simulink model "ARAI_Academy"  (R2020a)
settings: Solver=FixedStepDiscrete  StartTime=0.0  StopTime=10.0  FixedStep=0.02  RelTol=1e-3
InitFcn:
  | mbd_s32k_consistency_checks(bdroot(gcs));
undefined symbols (not defined in the file): Cells_in_Series, LQFP, Temp_in_Series, ts
libraries: hdlsllib x280, mbd_s32k1xx_ec_toolbox x39, simulink x3
(part 3 of 3)

== system ARAI_Academy/Subsystem15/Subsystem12/Subsystem8 ==
  u : Inport
  Bit Slice : hdlsllib/Logic and Bit Operations/Bit Slice  lidx=15  ridx=8
      settings: SourceProductBaseCode=SL
  Bit Slice1 : hdlsllib/Logic and Bit Operations/Bit Slice  lidx=7  ridx=0
      settings: SourceProductBaseCode=SL
  Mux : Mux  Inputs=2
  Out1 : Outport
  wires:
  Bit Slice/1 -> Mux/1
  u/1 -> Bit Slice/1, Bit Slice1/1
  Bit Slice1/1 -> Mux/2
  Mux/1 -> Out1/1

== system ARAI_Academy/Subsystem16/Subsystem12/Subsystem ==
  u : Inport
  Bit Slice : hdlsllib/Logic and Bit Operations/Bit Slice  lidx=15  ridx=8
      settings: SourceProductBaseCode=SL
  Bit Slice1 : hdlsllib/Logic and Bit Operations/Bit Slice  lidx=7  ridx=0
      settings: SourceProductBaseCode=SL
  Mux : Mux  Inputs=2
  Out1 : Outport
  wires:
  Bit Slice/1 -> Mux/1
  u/1 -> Bit Slice/1, Bit Slice1/1
  Bit Slice1/1 -> Mux/2
  Mux/1 -> Out1/1

== system ARAI_Academy/Subsystem16/Subsystem12/Subsystem1 ==
  u : Inport
  Bit Slice : hdlsllib/Logic and Bit Operations/Bit Slice  lidx=15  ridx=8
      settings: SourceProductBaseCode=SL
  Bit Slice1 : hdlsllib/Logic and Bit Operations/Bit Slice  lidx=7  ridx=0
      settings: SourceProductBaseCode=SL
  Mux : Mux  Inputs=2
  Out1 : Outport
  wires:
  Bit Slice/1 -> Mux/1
  u/1 -> Bit Slice/1, Bit Slice1/1
  Bit Slice1/1 -> Mux/2
  Mux/1 -> Out1/1

== system ARAI_Academy/Subsystem16/Subsystem12/Subsystem2 ==
  u : Inport
  Bit Slice : hdlsllib/Logic and Bit Operations/Bit Slice  lidx=15  ridx=8
      settings: SourceProductBaseCode=SL
  Bit Slice1 : hdlsllib/Logic and Bit Operations/Bit Slice  lidx=7  ridx=0
      settings: SourceProductBaseCode=SL
  Mux : Mux  Inputs=2
  Out1 : Outport
  wires:
  Bit Slice/1 -> Mux/1
  u/1 -> Bit Slice/1, Bit Slice1/1
  Bit Slice1/1 -> Mux/2
  Mux/1 -> Out1/1

== system ARAI_Academy/Subsystem16/Subsystem12/Subsystem3 ==
  u : Inport
  Bit Slice : hdlsllib/Logic and Bit Operations/Bit Slice  lidx=15  ridx=8
      settings: SourceProductBaseCode=SL
  Bit Slice1 : hdlsllib/Logic and Bit Operations/Bit Slice  lidx=7  ridx=0
      settings: SourceProductBaseCode=SL
  Mux : Mux  Inputs=2
  Out1 : Outport
  wires:
  Bit Slice/1 -> Mux/1
  u/1 -> Bit Slice/1, Bit Slice1/1
  Bit Slice1/1 -> Mux/2
  Mux/1 -> Out1/1

== system ARAI_Academy/Subsystem16/Subsystem12/Subsystem4 ==
  u : Inport
  Bit Slice : hdlsllib/Logic and Bit Operations/Bit Slice  lidx=15  ridx=8
      settings: SourceProductBaseCode=SL
  Bit Slice1 : hdlsllib/Logic and Bit Operations/Bit Slice  lidx=7  ridx=0
      settings: SourceProductBaseCode=SL
  Mux : Mux  Inputs=2
  Out1 : Outport
  wires:
  Bit Slice/1 -> Mux/1
  u/1 -> Bit Slice/1, Bit Slice1/1
  Bit Slice1/1 -> Mux/2
  Mux/1 -> Out1/1

== system ARAI_Academy/Subsystem16/Subsystem12/Subsystem5 ==
  u : Inport
  Bit Slice : hdlsllib/Logic and Bit Operations/Bit Slice  lidx=15  ridx=8
      settings: SourceProductBaseCode=SL
  Bit Slice1 : hdlsllib/Logic and Bit Operations/Bit Slice  lidx=7  ridx=0
      settings: SourceProductBaseCode=SL
  Mux : Mux  Inputs=2
  Out1 : Outport
  wires:
  Bit Slice/1 -> Mux/1
  u/1 -> Bit Slice/1, Bit Slice1/1
  Bit Slice1/1 -> Mux/2
  Mux/1 -> Out1/1

== system ARAI_Academy/Subsystem16/Subsystem12/Subsystem7 ==
  u : Inport
  Bit Slice : hdlsllib/Logic and Bit Operations/Bit Slice  lidx=15  ridx=8
      settings: SourceProductBaseCode=SL
  Bit Slice1 : hdlsllib/Logic and Bit Operations/Bit Slice  lidx=7  ridx=0
      settings: SourceProductBaseCode=SL
  Mux : Mux  Inputs=2
  Out1 : Outport
  wires:
  Mux/1 -> Out1/1
  Bit Slice1/1 -> Mux/2
  u/1 -> Bit Slice1/1, Bit Slice/1
  Bit Slice/1 -> Mux/1

== system ARAI_Academy/Subsystem16/Subsystem12/Subsystem8 ==
  u : Inport
  Bit Slice : hdlsllib/Logic and Bit Operations/Bit Slice  lidx=15  ridx=8
      settings: SourceProductBaseCode=SL
  Bit Slice1 : hdlsllib/Logic and Bit Operations/Bit Slice  lidx=7  ridx=0
      settings: SourceProductBaseCode=SL
  Mux : Mux  Inputs=2
  Out1 : Outport
  wires:
  Bit Slice/1 -> Mux/1
  u/1 -> Bit Slice/1, Bit Slice1/1
  Bit Slice1/1 -> Mux/2
  Mux/1 -> Out1/1

== system ARAI_Academy/Subsystem9/Subsystem/Subsystem ==
  u : Inport
  Bit Slice : hdlsllib/Logic and Bit Operations/Bit Slice  lidx=15  ridx=8
      settings: SourceProductBaseCode=SL
  Bit Slice1 : hdlsllib/Logic and Bit Operations/Bit Slice  lidx=7  ridx=0
      settings: SourceProductBaseCode=SL
  Mux : Mux  Inputs=2
  Out1 : Outport
  wires:
  Bit Slice/1 -> Mux/1
  u/1 -> Bit Slice/1, Bit Slice1/1
  Bit Slice1/1 -> Mux/2
  Mux/1 -> Out1/1

== system ARAI_Academy/Subsystem9/Subsystem/Subsystem1 ==
  u : Inport
  Bit Slice : hdlsllib/Logic and Bit Operations/Bit Slice  lidx=15  ridx=8
      settings: SourceProductBaseCode=SL
  Bit Slice1 : hdlsllib/Logic and Bit Operations/Bit Slice  lidx=7  ridx=0
      settings: SourceProductBaseCode=SL
  Mux : Mux  Inputs=2
  Out1 : Outport
  wires:
  Bit Slice/1 -> Mux/1
  u/1 -> Bit Slice/1, Bit Slice1/1
  Bit Slice1/1 -> Mux/2
  Mux/1 -> Out1/1

== system ARAI_Academy/Subsystem9/Subsystem/Subsystem10 ==
  u : Inport
  Bit Slice : hdlsllib/Logic and Bit Operations/Bit Slice  lidx=15  ridx=8
      settings: SourceProductBaseCode=SL
  Bit Slice1 : hdlsllib/Logic and Bit Operations/Bit Slice  lidx=7  ridx=0
      settings: SourceProductBaseCode=SL
  Mux : Mux  Inputs=2
  Out1 : Outport
  wires:
  Bit Slice/1 -> Mux/1
  u/1 -> Bit Slice/1, Bit Slice1/1
  Bit Slice1/1 -> Mux/2
  Mux/1 -> Out1/1

== system ARAI_Academy/Subsystem9/Subsystem/Subsystem11 ==
  u : Inport
  Bit Slice : hdlsllib/Logic and Bit Operations/Bit Slice  lidx=15  ridx=8
      settings: SourceProductBaseCode=SL
  Bit Slice1 : hdlsllib/Logic and Bit Operations/Bit Slice  lidx=7  ridx=0
      settings: SourceProductBaseCode=SL
  Mux : Mux  Inputs=2
  Out1 : Outport
  wires:
  Mux/1 -> Out1/1
  Bit Slice1/1 -> Mux/2
  u/1 -> Bit Slice1/1, Bit Slice/1
  Bit Slice/1 -> Mux/1

== system ARAI_Academy/Subsystem9/Subsystem/Subsystem12 ==
  u : Inport
  Bit Slice : hdlsllib/Logic and Bit Operations/Bit Slice  lidx=15  ridx=8
      settings: SourceProductBaseCode=SL
  Bit Slice1 : hdlsllib/Logic and Bit Operations/Bit Slice  lidx=7  ridx=0
      settings: SourceProductBaseCode=SL
  Mux : Mux  Inputs=2
  Out1 : Outport
  wires:
  Bit Slice/1 -> Mux/1
  u/1 -> Bit Slice/1, Bit Slice1/1
  Bit Slice1/1 -> Mux/2
  Mux/1 -> Out1/1

== system ARAI_Academy/Subsystem9/Subsystem/Subsystem13 ==
  u : Inport
  Bit Slice : hdlsllib/Logic and Bit Operations/Bit Slice  lidx=15  ridx=8
      settings: SourceProductBaseCode=SL
  Bit Slice1 : hdlsllib/Logic and Bit Operations/Bit Slice  lidx=7  ridx=0
      settings: SourceProductBaseCode=SL
  Mux : Mux  Inputs=2
  Out1 : Outport
  wires:
  Mux/1 -> Out1/1
  Bit Slice1/1 -> Mux/2
  u/1 -> Bit Slice1/1, Bit Slice/1
  Bit Slice/1 -> Mux/1

== system ARAI_Academy/Subsystem9/Subsystem/Subsystem14 ==
  u : Inport
  Bit Slice : hdlsllib/Logic and Bit Operations/Bit Slice  lidx=15  ridx=8
      settings: SourceProductBaseCode=SL
  Bit Slice1 : hdlsllib/Logic and Bit Operations/Bit Slice  lidx=7  ridx=0
      settings: SourceProductBaseCode=SL
  Mux : Mux  Inputs=2
  Out1 : Outport
  wires:
  Bit Slice/1 -> Mux/1
  u/1 -> Bit Slice/1, Bit Slice1/1
  Bit Slice1/1 -> Mux/2
  Mux/1 -> Out1/1

== system ARAI_Academy/Subsystem9/Subsystem/Subsystem15 ==
  u : Inport
  Bit Slice : hdlsllib/Logic and Bit Operations/Bit Slice  lidx=15  ridx=8
      settings: SourceProductBaseCode=SL
  Bit Slice1 : hdlsllib/Logic and Bit Operations/Bit Slice  lidx=7  ridx=0
      settings: SourceProductBaseCode=SL
  Mux : Mux  Inputs=2
  Out1 : Outport
  wires:
  Mux/1 -> Out1/1
  Bit Slice1/1 -> Mux/2
  u/1 -> Bit Slice1/1, Bit Slice/1
  Bit Slice/1 -> Mux/1

== system ARAI_Academy/Subsystem9/Subsystem/Subsystem2 ==
  u : Inport
  Bit Slice : hdlsllib/Logic and Bit Operations/Bit Slice  lidx=15  ridx=8
      settings: SourceProductBaseCode=SL
  Bit Slice1 : hdlsllib/Logic and Bit Operations/Bit Slice  lidx=7  ridx=0
      settings: SourceProductBaseCode=SL
  Mux : Mux  Inputs=2
  Out1 : Outport
  wires:
  Bit Slice/1 -> Mux/1
  u/1 -> Bit Slice/1, Bit Slice1/1
  Bit Slice1/1 -> Mux/2
  Mux/1 -> Out1/1

== system ARAI_Academy/Subsystem9/Subsystem/Subsystem3 ==
  u : Inport
  Bit Slice : hdlsllib/Logic and Bit Operations/Bit Slice  lidx=15  ridx=8
      settings: SourceProductBaseCode=SL
  Bit Slice1 : hdlsllib/Logic and Bit Operations/Bit Slice  lidx=7  ridx=0
      settings: SourceProductBaseCode=SL
  Mux : Mux  Inputs=2
  Out1 : Outport
  wires:
  Bit Slice/1 -> Mux/1
  u/1 -> Bit Slice/1, Bit Slice1/1
  Bit Slice1/1 -> Mux/2
  Mux/1 -> Out1/1

== system ARAI_Academy/Subsystem9/Subsystem/Subsystem4 ==
  u : Inport
  Bit Slice : hdlsllib/Logic and Bit Operations/Bit Slice  lidx=15  ridx=8
      settings: SourceProductBaseCode=SL
  Bit Slice1 : hdlsllib/Logic and Bit Operations/Bit Slice  lidx=7  ridx=0
      settings: SourceProductBaseCode=SL
  Mux : Mux  Inputs=2
  Out1 : Outport
  wires:
  Bit Slice/1 -> Mux/1
  u/1 -> Bit Slice/1, Bit Slice1/1
  Bit Slice1/1 -> Mux/2
  Mux/1 -> Out1/1

== system ARAI_Academy/Subsystem9/Subsystem/Subsystem5 ==
  u : Inport
  Bit Slice : hdlsllib/Logic and Bit Operations/Bit Slice  lidx=15  ridx=8
      settings: SourceProductBaseCode=SL
  Bit Slice1 : hdlsllib/Logic and Bit Operations/Bit Slice  lidx=7  ridx=0
      settings: SourceProductBaseCode=SL
  Mux : Mux  Inputs=2
  Out1 : Outport
  wires:
  Bit Slice/1 -> Mux/1
  u/1 -> Bit Slice/1, Bit Slice1/1
  Bit Slice1/1 -> Mux/2
  Mux/1 -> Out1/1

== system ARAI_Academy/Subsystem9/Subsystem/Subsystem6 ==
  u : Inport
  Bit Slice : hdlsllib/Logic and Bit Operations/Bit Slice  lidx=15  ridx=8
      settings: SourceProductBaseCode=SL
  Bit Slice1 : hdlsllib/Logic and Bit Operations/Bit Slice  lidx=7  ridx=0
      settings: SourceProductBaseCode=SL
  Mux : Mux  Inputs=2
  Out1 : Outport
  wires:
  Bit Slice/1 -> Mux/1
  u/1 -> Bit Slice/1, Bit Slice1/1
  Bit Slice1/1 -> Mux/2
  Mux/1 -> Out1/1

== system ARAI_Academy/Subsystem9/Subsystem/Subsystem7 ==
  u : Inport
  Bit Slice : hdlsllib/Logic and Bit Operations/Bit Slice  lidx=15  ridx=8
      settings: SourceProductBaseCode=SL
  Bit Slice1 : hdlsllib/Logic and Bit Operations/Bit Slice  lidx=7  ridx=0
      settings: SourceProductBaseCode=SL
  Mux : Mux  Inputs=2
  Out1 : Outport
  wires:
  Mux/1 -> Out1/1
  Bit Slice1/1 -> Mux/2
  u/1 -> Bit Slice1/1, Bit Slice/1
  Bit Slice/1 -> Mux/1

== system ARAI_Academy/Subsystem9/Subsystem/Subsystem8 ==
  u : Inport
  Bit Slice : hdlsllib/Logic and Bit Operations/Bit Slice  lidx=15  ridx=8
      settings: SourceProductBaseCode=SL
  Bit Slice1 : hdlsllib/Logic and Bit Operations/Bit Slice  lidx=7  ridx=0
      settings: SourceProductBaseCode=SL
  Mux : Mux  Inputs=2
  Out1 : Outport
  wires:
  Bit Slice/1 -> Mux/1
  u/1 -> Bit Slice/1, Bit Slice1/1
  Bit Slice1/1 -> Mux/2
  Mux/1 -> Out1/1

== system ARAI_Academy/Subsystem9/Subsystem/Subsystem9 ==
  u : Inport
  Bit Slice : hdlsllib/Logic and Bit Operations/Bit Slice  lidx=15  ridx=8
      settings: SourceProductBaseCode=SL
  Bit Slice1 : hdlsllib/Logic and Bit Operations/Bit Slice  lidx=7  ridx=0
      settings: SourceProductBaseCode=SL
  Mux : Mux  Inputs=2
  Out1 : Outport
  wires:
  Mux/1 -> Out1/1
  Bit Slice1/1 -> Mux/2
  u/1 -> Bit Slice1/1, Bit Slice/1
  Bit Slice/1 -> Mux/1

== system ARAI_Academy/TNS/ADC/ADC_01 ==
  ADC_Config : mbd_s32k1xx_ec_toolbox/Motor Control Blocks/ADC Blocks/ADC_Config  instance=0  mode=12-bit conversion  smplts=2  adiclk=alternate clock 1  adiv=input clock  show_adv_opts=on  pretrgsel=PDB pre-trigger  swpretrg=Disabled  adtrg=software  trgsel=TRGMUX output  refsel=Vrefh and Vrefl  supply_monitoring=off  acfe=off  acfgt=off  acren=off  cv1=0  cv2=0  adco=off  avge=off  avgs=4 samples

== system ARAI_Academy/TNS/ADC/ADC_02 ==
  ADC_Config : mbd_s32k1xx_ec_toolbox/Motor Control Blocks/ADC Blocks/ADC_Config  instance=1  mode=12-bit conversion  smplts=2  adiclk=alternate clock 1  adiv=input clock  show_adv_opts=on  pretrgsel=PDB pre-trigger  swpretrg=Disabled  adtrg=software  trgsel=TRGMUX output  refsel=Vrefh and Vrefl  supply_monitoring=off  acfe=off  acfgt=off  acren=off  cv1=0  cv2=0  adco=off  avge=off  avgs=4 samples

== system ARAI_Academy/TNS/CAN/CAN_01 ==
  FCAN_Config : mbd_s32k1xx_ec_toolbox/Communication Blocks/CAN Blocks/FCAN_Config  Priority=1  can_instance=0  can_mode=Normal mode  can_max_num_mb=32  can_rx=PTE4: [CAN0_RX | CAN Rx channel]  can_tx=PTE5: [CAN0_TX | CAN Tx Channel]  show_adv_opts=on  can_clk_src=Peripheral clock  can_clk_freq=80 MHz  bitrate_to_time_seg=on  bitrate=500  sample_point=80  real_bitrate=500  real_sample_point=80  prop_delay=250  bus_length=1  tq=200.0  time_quanta=10  can_presdiv=16  can_propseg=3  can_pseg1=4  can_pseg2=2  can_rjw=2  cbt_bitrate=2000  cbt_sample_point=80  cbt_real_bitrate=2000  cbt_real_sample_point=80  cbt_tq=25.0  cbt_time_quanta=40  can_cbt_presdiv=3  can_cbt_propseg=6  can_cbt_pseg1=7  can_cbt_pseg2=7  can_cbt_rjw=3  can_fd_enable=off  can_payload=8  tdc_enable=off  tdc_offset=20  can_rxfifo_enable=off  can_num_id_filters=8  can_fifo_id_format=A  can_fifo_id_filter={'0x0', '0x0', '0x0', '0x0', '0x0', '0x0', '0x0', '0x0'}  can_pn_enable=off  can_wakeup_match=off  can_wakeup_timeout=off  can_timeout_en=off  can_match_timeout=1  can_multiple_matches_en=off  can_num_matches=1  can_idfilter_extendedid=off  can_idfilter_remoteframe=off  can_idfilter_type=Match exact  can_idfilter_id1=0  can_idfilter_id2=0  can_payloadfilter_enable=off  can_payloadfilter_dlclow=0  can_payloadfilter_dlchigh=0  can_payloadfilter_type=Match exact  can_payloadfilter_payload1_b0=0  can_payloadfilter_payload1_b1=0  can_payloadfilter_payload1_b2=0  can_payloadfilter_payload1_b3=0  can_payloadfilter_payload1_b4=0  can_payloadfilter_payload1_b5=0  can_payloadfilter_payload1_b6=0  can_payloadfilter_payload1_b7=0  can_payloadfilter_payload2_b0=0  can_payloadfilter_payload2_b1=0  can_payloadfilter_payload2_b2=0  can_payloadfilter_payload2_b3=0  can_payloadfilter_payload2_b4=0  can_payloadfilter_payload2_b5=0  can_payloadfilter_payload2_b6=0  can_payloadfilter_payload2_b7=0

== system ARAI_Academy/TNS/I2C/RTC//EEPROM ==
  LPI2C_Config : mbd_s32k1xx_ec_toolbox/Communication Blocks/I2C Blocks/LPI2C_Config  instance=0  mode=Master  opmode=Standard (up to 100 kbit/s)  bdr=400000  addr=1  is10bitaddr=off  sda=PTA2: [LPI2C0_SDA | LPI2C Data I/O]  scl=PTA3: [LPI2C0_SCL | LPI2C Clock I/O]

== stateflow chart ARAI_Academy/Chart ==
  state Standy_By
    en:P=0;
    C=0;
    D=0;
  state PreCharge
    en:P=1;
  state DisCharge
    en:P=0;
  state Charge
    en:P =0;
  state Transition
    en:P=1;
    C=1;
  state Transition1
    en:P=1;
    D=1;
  (default) -> Standy_By
  Charge -> Standy_By : [IGN==false]
  DisCharge -> Standy_By : [IGN==false]
  Standy_By -> PreCharge : [IGN==true]
  PreCharge -> Transition [order 1] : [after(3,sec)&&Charge==true]
  PreCharge -> Transition1 [order 2] : after(3,sec)
  Transition1 -> DisCharge : after(0.2,sec)
  Transition -> Charge : after(0.2,sec)
  data: IGN input; P output; C output; D output; Charge input

== stateflow chart ARAI_Academy/AFE_IN_SYS/Chart4 ==
  note: Note: The checksum value is 1 less than calculated checksum.
      | To calculate, enter the register address and data into calculator.
      | Link: http://easyonlineconverter.com/converters/checksum_converter.html
  state Tesdt
  state Initialize
    en:Next=false;
    en:CONFIG_UPDATE_0x0090();
  state Checksum8
    en:Checksum_0x92FA();
  state Checksum16
    en:Checksum_0x91EA();
  state CFETOFF_Pin
    en:Pin_Confi_0x92FA();
  state COEFF_a1
    en:Pin_Confi_0x91EA();
  state Checksum13
    en:Checksum_0x9335();
  state Balancing_Pin
    en:Pin_Confi_0x9335();
  state Cell_Balance_Interval
    en:Pin_Confi_0x9339();
  state Checksum4
    en:Checksum_0x9339();
  state Conf_exit
    en:EXIT_CFGUPDATE_0x9200();
  state Conf_enter
    en:Next=true;
  state CONFIG_UPDATE_0x0090 [function]
  state Pin_Confi_0x9335 [function]
  state Pin_Confi_0x9339 [function]
  state Checksum_0x9335 [function]
  state Checksum_0x9339 [function]
  state EXIT_CFGUPDATE_0x9200 [function]
  state Pin_Confi_0x91EA [function]
  state Pin_Confi_0x92FA [function]
  state Checksum_0x91EA [function]
  state Checksum_0x92FA [function]
  (default) -> Tesdt
  Tesdt -> Initialize : after(2,sec)
  Balancing_Pin -> Checksum13 : after(delay,sec)
  Checksum13 -> Cell_Balance_Interval : after(delay,sec)
  Cell_Balance_Interval -> Checksum4 : after(delay,sec)
  Initialize -> COEFF_a1 : after(delay,sec)
  COEFF_a1 -> Checksum16 : after(delay,sec)
  CFETOFF_Pin -> Checksum8 : after(delay,sec)
  Checksum16 -> CFETOFF_Pin : after(delay,sec)
  Checksum8 -> Balancing_Pin : after(delay,sec)
  Checksum4 -> Conf_exit : after(delay,sec)
  Conf_exit -> Conf_enter : after(delay,sec)
  data: delay input; Next output

== stateflow chart ARAI_Academy/TNS/Blink ==
  state A
  state A1
  (default) -> A
  A -> A1 : after(0.2,sec)
  A1 -> A : after(0.2,sec)
  data: A output boolean [0..1]
